simulink model "joitick_pruena"  (R2021a)
settings: Solver=VariableStepAuto  StartTime=0.0  StopTime=50  RelTol=1e-3
undefined symbols (not defined in the file): dt
libraries: aerolibanimutils x2
settings Model: Creator=facu_  LastModifiedBy=facu_

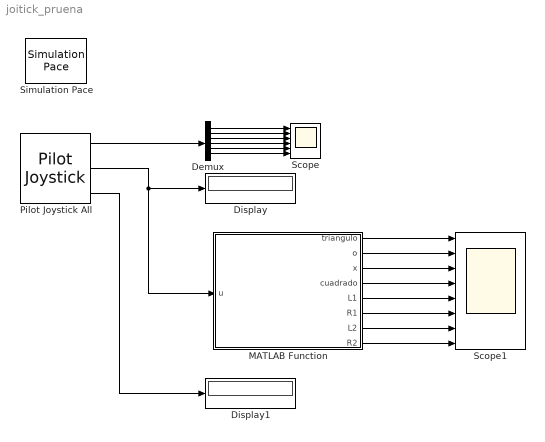
== system joitick_pruena ==
  Demux : Demux  Outputs=6
  Display : Display
  Display1 : Display
  MATLAB Function : MATLAB Function  TreatAsAtomicUnit=on
  Pilot Joystick All : aerolibanimutils/Pilot Joystick  JoystickID=Joystick1  OutputConfiguration=AllOutputs  SampleTime=1/30
  Scope : Scope  NumInputPorts=6
  Scope1 : Scope  NumInputPorts=8
  Simulation Pace : aerolibanimutils/Simulation Pace  SimulationPace=1  SleepMode=Auto  OutputPaceError=off  SampleTime=dt
  wires:
  Pilot Joystick All/1 -> Demux/1
  Demux/1 -> Scope/1
  Demux/2 -> Scope/2
  Demux/3 -> Scope/3
  Demux/4 -> Scope/4
  Demux/5 -> Scope/5
  Demux/6 -> Scope/6
  Pilot Joystick All/3 -> Display1/1
  Pilot Joystick All/2 -> MATLAB Function/1(u), Display/1
  MATLAB Function/1(triangulo) -> Scope1/1
  MATLAB Function/2(o) -> Scope1/2
  MATLAB Function/3(x) -> Scope1/3
  MATLAB Function/4(cuadrado) -> Scope1/4
  MATLAB Function/5(L1) -> Scope1/5
  MATLAB Function/6(R1) -> Scope1/6
  MATLAB Function/7(L2) -> Scope1/7
  MATLAB Function/8(R2) -> Scope1/8

== matlab function joitick_pruena/MATLAB Function ==
  data: triangulo output; o output; x output; cuadrado output; u input; L1 output; R1 output; L2 output; R2 output
function [triangulo, o, x, cuadrado, L1, R1, L2, R2] = buttonMap(u)
    triangulo = double(bitand(u, 1));
    
    u = bitshift(u, -1);
    o = double(bitand(u, 1));
    
    u = bitshift(u, -1);
    x = double(bitand(u, 1));
    
    u = bitshift(u, -1);
    cuadrado = double(bitand(u, 1));
    
    u = bitshift(u, -1);
    L1 = double(bitand(u, 1));
    
    u = bitshift(u, -1);
    R1 = double(not(bitand(u, 1)));
    
    u = bitshift(u, -1);
    L2 = double(bitand(u, 1));
    
    u = bitshift(u, -1);
    R2 = double(bitand(u, 1));
end
